simulink model "Mecanum_Mfunction_SM"  (R2022b)
settings: Solver=FixedStepAuto  StartTime=0.0  StopTime=20  FixedStep=0.001  RelTol=1e-3
values from neighbouring files (symbols this model uses):
  Cm = 0    [Mecanum_parameter_Mfunction_PI.m]    (also in Mecanum_parameter_Mfunction_PID.m; Mecanum_parameter_Mfunction_SM.m)
  Jm = 0    [Mecanum_parameter_Mfunction_PI.m]    (also in Mecanum_parameter_Mfunction_PID.m = 1.55e-06; Mecanum_parameter_Mfunction_SM.m)
  Kb = Kt    (= 230)    [Mecanum_parameter_Mfunction_PI.m]    (also in Mecanum_parameter_Mfunction_PID.m; Mecanum_parameter_Mfunction_SM.m)
  Kf = 0    [Mecanum_parameter_Mfunction_PI.m]    (also in Mecanum_parameter_Mfunction_PID.m; Mecanum_parameter_Mfunction_SM.m)
  Kt = 230    [Mecanum_parameter_Mfunction_PI.m]    (also in Mecanum_parameter_Mfunction_PID.m; Mecanum_parameter_Mfunction_SM.m)
  La = 0.39*10^-3    (= 0.00039)    [Mecanum_parameter_Mfunction_PI.m]    (also in Mecanum_parameter_Mfunction_PID.m; Mecanum_parameter_Mfunction_SM.m)
  N = N_motor * N_wheel    (= 10)    [Mecanum_parameter_Mfunction_PI.m]    (also in Mecanum_parameter_Mfunction_PID.m; Mecanum_parameter_Mfunction_SM.m)
  Ra = 0.38    [Mecanum_parameter_Mfunction_PI.m]    (also in Mecanum_parameter_Mfunction_PID.m; Mecanum_parameter_Mfunction_SM.m)
libraries: simulink x2
settings Model: Creator=HONG  LastModifiedBy=CSPLAB
settings SolverCC: AlgebraicLoopSolver=TrustRegion
settings DataIOCC: ReturnWorkspaceOutputs=off
settings DebuggingCC: UnconnectedInputMsg=warning  UnconnectedOutputMsg=warning  UnconnectedLineMsg=warning  SFMachineParentedDataDiag=warning  ArithmeticOperatorsInVariantConditions=warning
settings ModelReferenceCC: EnableRefExpFcnMdlSchedulingChecks=on
settings SFSimCC: CustomCodeUndefinedFunction=UseInterfaceOnly

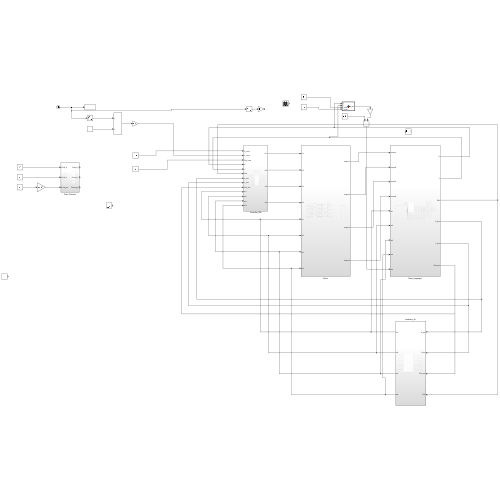
[thumbnail: Simulink's stored preview of the top-level diagram]
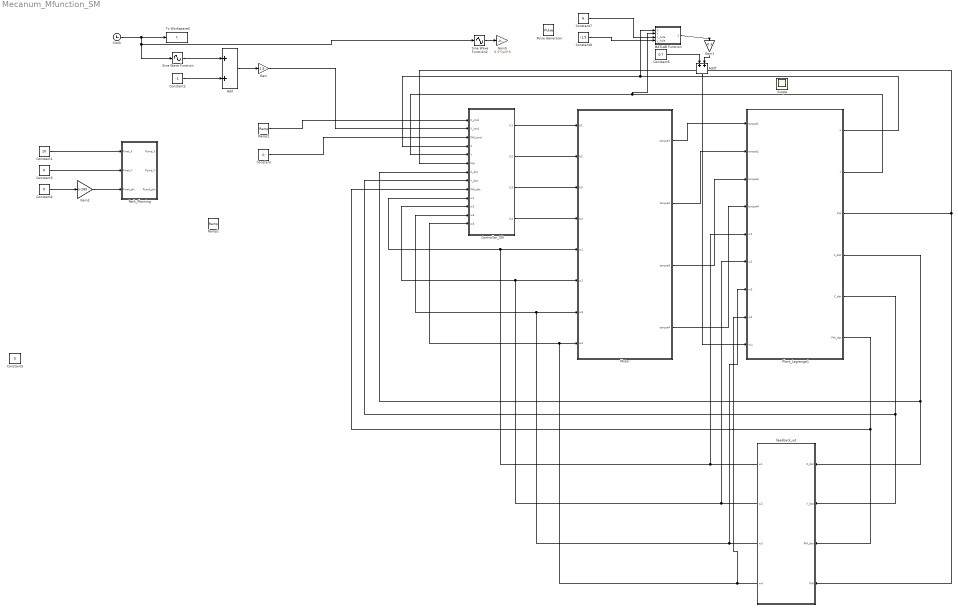
== system Mecanum_Mfunction_SM ==
  Add : Sum
  Add7 : Sum
  Clock : Clock
  Constant{,3..5} (4 alike) : Constant  Value=0
  Constant1 : Constant  Value=10
  Constant2 : Constant  Value=-1
  Constant6 : Constant  Value=0.7
  Constant7 : Constant  Value=6
  Constant8 : Constant  Value=-1.5
  Controller_SM : Subsystem
  Gain : Gain  Gain=1.5
  Gain1 : Gain  Gain=-0.3
  Gain2 : Gain  Gain=pi/180
  Gain5 : Gain  Gain=0.5*1e3*0
  MATLAB Function : MATLAB Function  TreatAsAtomicUnit=on
  Motor : Subsystem
  Path_Planning : Subsystem
  Plant_Lagrange1 : Subsystem
  Pulse Generator : DiscretePulseGenerator  PulseType=Time based  Period=10  PulseWidth=5
  Ramp1 : simulink/Sources/Ramp  slope=1.5  start=0  InitialOutput=0
  Ramp2 : simulink/Sources/Ramp  slope=0.5  start=0  InitialOutput=0
  Scope : Scope
  Sine Wave Function : Sin  TimeSource=Use external signal  Frequency=pi/8  Phase=pi/2  SampleTime=0
  Sine Wave Function2 : Sin  TimeSource=Use external signal  Frequency=pi/0.5  Phase=pi/2  SampleTime=0
  To Workspace5 : ToWorkspace  VariableName=t  SampleTime=-1
  feedback_w1 : Subsystem
  wires:
  Plant_Lagrange1/4(X_dot) -> Controller_SM/7(X_dot), feedback_w1/1(X_dot)
  Plant_Lagrange1/5(Y_dot) -> Controller_SM/8(Y_dot), feedback_w1/2(Y_dot)
  Plant_Lagrange1/6(PHI_dot) -> Controller_SM/9(PHI_dot), feedback_w1/3(PHI_dot)
  Plant_Lagrange1/3(PHI) -> feedback_w1/4(PHI), Controller_SM/6(PHI)
  feedback_w1/1(w1) -> Controller_SM/10(w1), Motor/5(w1), Plant_Lagrange1/5(w1)
  feedback_w1/2(w2) -> Plant_Lagrange1/6(w2), Controller_SM/11(w2), Motor/6(w2)
  feedback_w1/3(w3) -> Plant_Lagrange1/7(w3), Controller_SM/12(w3), Motor/7(w3)
  feedback_w1/4(w4) -> Plant_Lagrange1/8(w4), Controller_SM/13(w4), Motor/8(w4)
  Plant_Lagrange1/1(X) -> MATLAB Function/1(X), Controller_SM/4(X)
  Plant_Lagrange1/2(Y) -> MATLAB Function/2(Y), Controller_SM/5(Y)
  Clock/1 -> Sine Wave Function/1, Sine Wave Function2/1, To Workspace5/1
  Controller_SM/1(U1) -> Motor/1(U1)
  Controller_SM/2(U2) -> Motor/2(U2)
  Controller_SM/3(U3) -> Motor/3(U3)
  Controller_SM/4(U4) -> Motor/4(U4)
  Constant/1 -> Controller_SM/3(PHI_cmd)
  Constant2/1 -> Add/2
  Add/1 -> Gain/1
  Sine Wave Function/1 -> Add/1
  Constant1/1 -> Path_Planning/1(Final_X)
  Constant3/1 -> Path_Planning/2(Final_Y)
  Gain2/1 -> Path_Planning/3(Final_phi)
  Constant4/1 -> Gain2/1
  Gain/1 -> Controller_SM/2(Y_cmd)
  Ramp2/1 -> Controller_SM/1(X_cmd)
  Sine Wave Function2/1 -> Gain5/1
  Gain1/1 -> Add7/2
  Motor/2(torque2) -> Plant_Lagrange1/2(torque2)
  Motor/1(torque1) -> Plant_Lagrange1/1(torque1)
  Motor/3(torque3) -> Plant_Lagrange1/3(torque3)
  Motor/4(torque4) -> Plant_Lagrange1/4(torque4)
  Add7/1 -> Plant_Lagrange1/9(mu)
  Constant6/1 -> Add7/1
  MATLAB Function/1(Delta_mu) -> Gain1/1
  Constant7/1 -> MATLAB Function/3(x_hole)
  Constant8/1 -> MATLAB Function/4(y_hole)

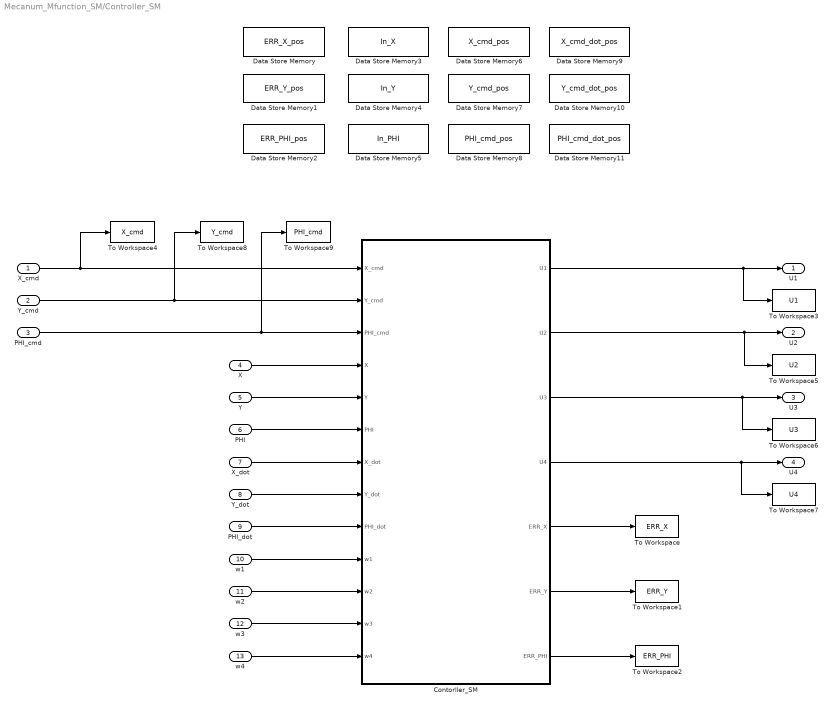
== system Mecanum_Mfunction_SM/Controller_SM ==
  X_cmd : Inport
  Y_cmd : Inport  Port=2
  PHI_cmd : Inport  Port=3
  X : Inport  Port=4
  Y : Inport  Port=5
  PHI : Inport  Port=6
  X_dot : Inport  Port=7
  Y_dot : Inport  Port=8
  PHI_dot : Inport  Port=9
  w1 : Inport  Port=10
  w2 : Inport  Port=11
  w3 : Inport  Port=12
  w4 : Inport  Port=13
  "Contorller_SM " : MATLAB Function  TreatAsAtomicUnit=on
  Data Store Memory : DataStoreMemory  DataStoreName=ERR_X_pos  ReadBeforeWriteMsg=warning  WriteAfterWriteMsg=warning  WriteAfterReadMsg=warning  ShowAdditionalParam=off  OutDataTypeStr=double
  Data Store Memory1 : DataStoreMemory  DataStoreName=ERR_Y_pos  ReadBeforeWriteMsg=warning  WriteAfterWriteMsg=warning  WriteAfterReadMsg=warning  ShowAdditionalParam=off  OutDataTypeStr=double
  Data Store Memory10 : DataStoreMemory  DataStoreName=Y_cmd_dot_pos  ReadBeforeWriteMsg=warning  WriteAfterWriteMsg=warning  WriteAfterReadMsg=warning  ShowAdditionalParam=off  OutDataTypeStr=double
  Data Store Memory11 : DataStoreMemory  DataStoreName=PHI_cmd_dot_pos  ReadBeforeWriteMsg=warning  WriteAfterWriteMsg=warning  WriteAfterReadMsg=warning  ShowAdditionalParam=off  OutDataTypeStr=double
  Data Store Memory2 : DataStoreMemory  DataStoreName=ERR_PHI_pos  ReadBeforeWriteMsg=warning  WriteAfterWriteMsg=warning  WriteAfterReadMsg=warning  ShowAdditionalParam=off  OutDataTypeStr=double
  Data Store Memory3 : DataStoreMemory  DataStoreName=In_X  ReadBeforeWriteMsg=warning  WriteAfterWriteMsg=warning  WriteAfterReadMsg=warning  ShowAdditionalParam=off  OutDataTypeStr=double
  Data Store Memory4 : DataStoreMemory  DataStoreName=In_Y  ReadBeforeWriteMsg=warning  WriteAfterWriteMsg=warning  WriteAfterReadMsg=warning  ShowAdditionalParam=off  OutDataTypeStr=double
  Data Store Memory5 : DataStoreMemory  DataStoreName=In_PHI  ReadBeforeWriteMsg=warning  WriteAfterWriteMsg=warning  WriteAfterReadMsg=warning  ShowAdditionalParam=off  OutDataTypeStr=double
  Data Store Memory6 : DataStoreMemory  DataStoreName=X_cmd_pos  ReadBeforeWriteMsg=warning  WriteAfterWriteMsg=warning  WriteAfterReadMsg=warning  ShowAdditionalParam=off  OutDataTypeStr=double
  Data Store Memory7 : DataStoreMemory  DataStoreName=Y_cmd_pos  ReadBeforeWriteMsg=warning  WriteAfterWriteMsg=warning  WriteAfterReadMsg=warning  ShowAdditionalParam=off  OutDataTypeStr=double
  Data Store Memory8 : DataStoreMemory  DataStoreName=PHI_cmd_pos  ReadBeforeWriteMsg=warning  WriteAfterWriteMsg=warning  WriteAfterReadMsg=warning  ShowAdditionalParam=off  OutDataTypeStr=double
  Data Store Memory9 : DataStoreMemory  DataStoreName=X_cmd_dot_pos  ReadBeforeWriteMsg=warning  WriteAfterWriteMsg=warning  WriteAfterReadMsg=warning  ShowAdditionalParam=off  OutDataTypeStr=double
  To Workspace : ToWorkspace  VariableName=ERR_X  SampleTime=-1
  To Workspace1 : ToWorkspace  VariableName=ERR_Y  SampleTime=-1
  To Workspace2 : ToWorkspace  VariableName=ERR_PHI  SampleTime=-1
  To Workspace3 : ToWorkspace  VariableName=U1  SampleTime=-1
  To Workspace4 : ToWorkspace  VariableName=X_cmd  SampleTime=-1
  To Workspace5 : ToWorkspace  VariableName=U2  SampleTime=-1
  To Workspace6 : ToWorkspace  VariableName=U3  SampleTime=-1
  To Workspace7 : ToWorkspace  VariableName=U4  SampleTime=-1
  To Workspace8 : ToWorkspace  VariableName=Y_cmd  SampleTime=-1
  To Workspace9 : ToWorkspace  VariableName=PHI_cmd  SampleTime=-1
  U1 : Outport  VectorParamsAs1DForOutWhenUnconnected=off
  U2 : Outport  Port=2  VectorParamsAs1DForOutWhenUnconnected=off
  U3 : Outport  Port=3  VectorParamsAs1DForOutWhenUnconnected=off
  U4 : Outport  Port=4  VectorParamsAs1DForOutWhenUnconnected=off
  wires:
  "Contorller_SM "/4(U4) -> To Workspace7/1, U4/1
  "Contorller_SM "/3(U3) -> To Workspace6/1, U3/1
  "Contorller_SM "/2(U2) -> To Workspace5/1, U2/1
  "Contorller_SM "/1(U1) -> U1/1, To Workspace3/1
  w4/1 -> "Contorller_SM "/13(w4)
  w3/1 -> "Contorller_SM "/12(w3)
  w2/1 -> "Contorller_SM "/11(w2)
  w1/1 -> "Contorller_SM "/10(w1)
  PHI_dot/1 -> "Contorller_SM "/9(PHI_dot)
  Y_dot/1 -> "Contorller_SM "/8(Y_dot)
  X_dot/1 -> "Contorller_SM "/7(X_dot)
  PHI/1 -> "Contorller_SM "/6(PHI)
  Y/1 -> "Contorller_SM "/5(Y)
  X/1 -> "Contorller_SM "/4(X)
  PHI_cmd/1 -> To Workspace9/1, "Contorller_SM "/3(PHI_cmd)
  Y_cmd/1 -> To Workspace8/1, "Contorller_SM "/2(Y_cmd)
  X_cmd/1 -> To Workspace4/1, "Contorller_SM "/1(X_cmd)
  "Contorller_SM "/5(ERR_X) -> To Workspace/1
  "Contorller_SM "/7(ERR_PHI) -> To Workspace2/1
  "Contorller_SM "/6(ERR_Y) -> To Workspace1/1

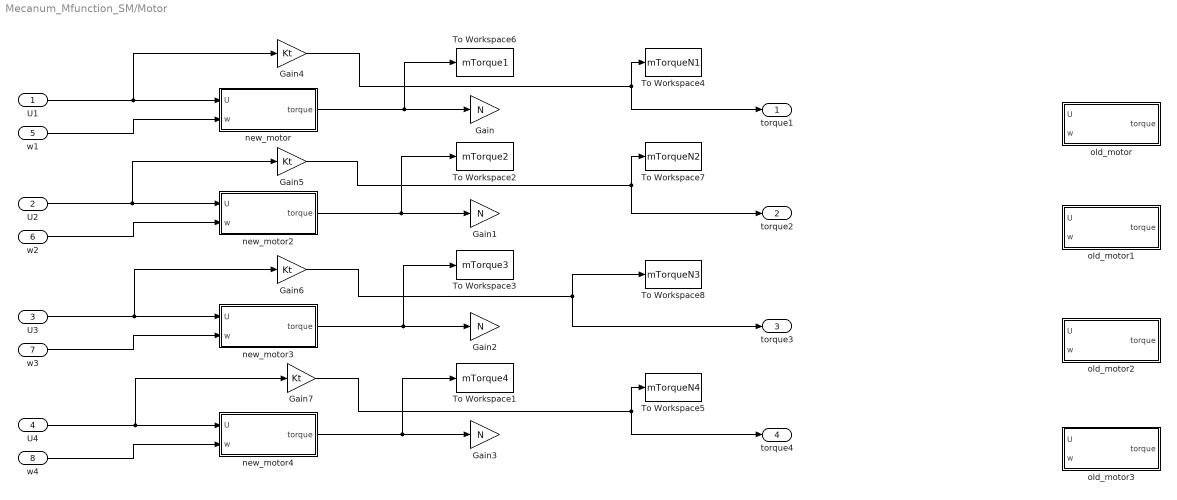
== system Mecanum_Mfunction_SM/Motor ==
  U1 : Inport
  U2 : Inport  Port=2
  U3 : Inport  Port=3
  U4 : Inport  Port=4
  w1 : Inport  Port=5
  w2 : Inport  Port=6
  w3 : Inport  Port=7
  w4 : Inport  Port=8
  Gain{,1..3} (4 alike) : Gain  Gain=N
  Gain{4..7} (4 alike) : Gain  Gain=Kt
  To Workspace1 : ToWorkspace  VariableName=mTorque4  SampleTime=-1
  To Workspace2 : ToWorkspace  VariableName=mTorque2  SampleTime=-1
  To Workspace3 : ToWorkspace  VariableName=mTorque3  SampleTime=-1
  To Workspace4 : ToWorkspace  VariableName=mTorqueN1  SampleTime=-1
  To Workspace5 : ToWorkspace  VariableName=mTorqueN4  SampleTime=-1
  To Workspace6 : ToWorkspace  VariableName=mTorque1  SampleTime=-1
  To Workspace7 : ToWorkspace  VariableName=mTorqueN2  SampleTime=-1
  To Workspace8 : ToWorkspace  VariableName=mTorqueN3  SampleTime=-1
  new_motor : Subsystem
  new_motor2 : Subsystem
  new_motor3 : Subsystem
  new_motor4 : Subsystem
  old_motor : Subsystem
  old_motor1 : Subsystem
  old_motor2 : Subsystem
  old_motor3 : Subsystem
  torque1 : Outport  VectorParamsAs1DForOutWhenUnconnected=off
  torque2 : Outport  Port=2  VectorParamsAs1DForOutWhenUnconnected=off
  torque3 : Outport  Port=3  VectorParamsAs1DForOutWhenUnconnected=off
  torque4 : Outport  Port=4  VectorParamsAs1DForOutWhenUnconnected=off
  wires:
  U1/1 -> Gain4/1, new_motor/1(U)
  w1/1 -> new_motor/2(w)
  w2/1 -> new_motor2/2(w)
  U2/1 -> Gain5/1, new_motor2/1(U)
  U3/1 -> Gain6/1, new_motor3/1(U)
  w3/1 -> new_motor3/2(w)
  U4/1 -> Gain7/1, new_motor4/1(U)
  w4/1 -> new_motor4/2(w)
  new_motor/1(torque) -> To Workspace6/1, Gain/1
  new_motor2/1(torque) -> To Workspace2/1, Gain1/1
  new_motor3/1(torque) -> To Workspace3/1, Gain2/1
  new_motor4/1(torque) -> Gain3/1, To Workspace1/1
  Gain4/1 -> To Workspace4/1, torque1/1
  Gain7/1 -> To Workspace5/1, torque4/1
  Gain6/1 -> To Workspace8/1, torque3/1
  Gain5/1 -> To Workspace7/1, torque2/1

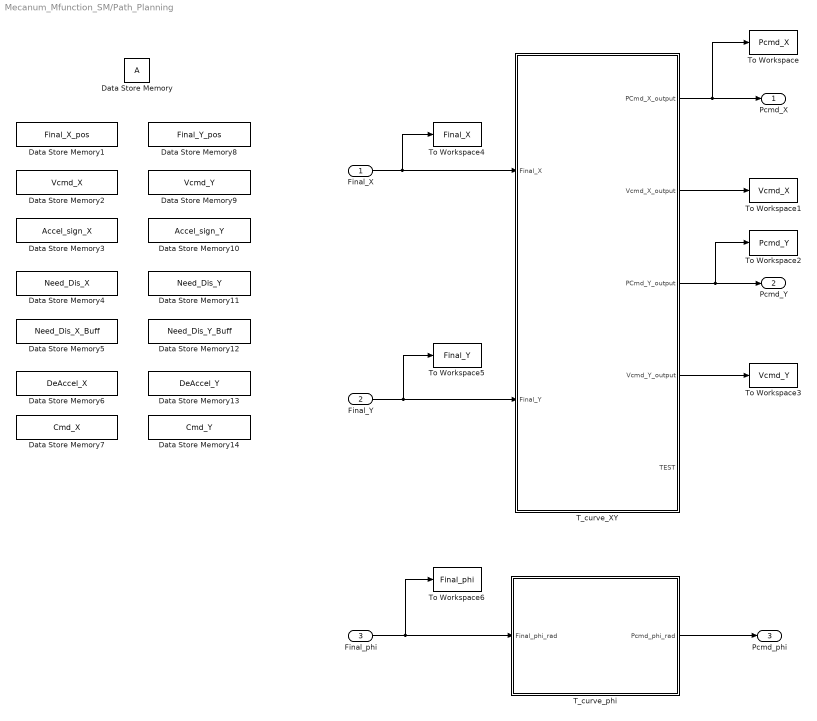
== system Mecanum_Mfunction_SM/Path_Planning ==
  Final_X : Inport
  Final_Y : Inport  Port=2
  Final_phi : Inport  Port=3
  Data Store Memory : DataStoreMemory  ReadBeforeWriteMsg=warning  WriteAfterWriteMsg=warning  WriteAfterReadMsg=warning  ShowAdditionalParam=off  OutDataTypeStr=double
  Data Store Memory1 : DataStoreMemory  DataStoreName=Final_X_pos  ReadBeforeWriteMsg=warning  WriteAfterWriteMsg=warning  WriteAfterReadMsg=warning  ShowAdditionalParam=off  OutDataTypeStr=double
  Data Store Memory10 : DataStoreMemory  DataStoreName=Accel_sign_Y  ReadBeforeWriteMsg=warning  WriteAfterWriteMsg=warning  WriteAfterReadMsg=warning  ShowAdditionalParam=off  OutDataTypeStr=double
  Data Store Memory11 : DataStoreMemory  DataStoreName=Need_Dis_Y  ReadBeforeWriteMsg=warning  WriteAfterWriteMsg=warning  WriteAfterReadMsg=warning  ShowAdditionalParam=off  OutDataTypeStr=double
  Data Store Memory12 : DataStoreMemory  DataStoreName=Need_Dis_Y_Buff  ReadBeforeWriteMsg=warning  WriteAfterWriteMsg=warning  WriteAfterReadMsg=warning  ShowAdditionalParam=off  OutDataTypeStr=double
  Data Store Memory13 : DataStoreMemory  DataStoreName=DeAccel_Y  ReadBeforeWriteMsg=warning  WriteAfterWriteMsg=warning  WriteAfterReadMsg=warning  ShowAdditionalParam=off  OutDataTypeStr=double
  Data Store Memory14 : DataStoreMemory  DataStoreName=Cmd_Y  ReadBeforeWriteMsg=warning  WriteAfterWriteMsg=warning  WriteAfterReadMsg=warning  ShowAdditionalParam=off  OutDataTypeStr=double
  Data Store Memory2 : DataStoreMemory  DataStoreName=Vcmd_X  ReadBeforeWriteMsg=warning  WriteAfterWriteMsg=warning  WriteAfterReadMsg=warning  ShowAdditionalParam=off  OutDataTypeStr=double
  Data Store Memory3 : DataStoreMemory  DataStoreName=Accel_sign_X  ReadBeforeWriteMsg=warning  WriteAfterWriteMsg=warning  WriteAfterReadMsg=warning  ShowAdditionalParam=off  OutDataTypeStr=double
  Data Store Memory4 : DataStoreMemory  DataStoreName=Need_Dis_X  ReadBeforeWriteMsg=warning  WriteAfterWriteMsg=warning  WriteAfterReadMsg=warning  ShowAdditionalParam=off  OutDataTypeStr=double
  Data Store Memory5 : DataStoreMemory  DataStoreName=Need_Dis_X_Buff  ReadBeforeWriteMsg=warning  WriteAfterWriteMsg=warning  WriteAfterReadMsg=warning  ShowAdditionalParam=off  OutDataTypeStr=double
  Data Store Memory6 : DataStoreMemory  DataStoreName=DeAccel_X  ReadBeforeWriteMsg=warning  WriteAfterWriteMsg=warning  WriteAfterReadMsg=warning  ShowAdditionalParam=off  OutDataTypeStr=double
  Data Store Memory7 : DataStoreMemory  DataStoreName=Cmd_X  ReadBeforeWriteMsg=warning  WriteAfterWriteMsg=warning  WriteAfterReadMsg=warning  ShowAdditionalParam=off  OutDataTypeStr=double
  Data Store Memory8 : DataStoreMemory  DataStoreName=Final_Y_pos  ReadBeforeWriteMsg=warning  WriteAfterWriteMsg=warning  WriteAfterReadMsg=warning  ShowAdditionalParam=off  OutDataTypeStr=double
  Data Store Memory9 : DataStoreMemory  DataStoreName=Vcmd_Y  ReadBeforeWriteMsg=warning  WriteAfterWriteMsg=warning  WriteAfterReadMsg=warning  ShowAdditionalParam=off  OutDataTypeStr=double
  "T_curve_XY " : MATLAB Function  TreatAsAtomicUnit=on
  T_curve_phi : Subsystem
  To Workspace : ToWorkspace  VariableName=Pcmd_X  SampleTime=-1
  To Workspace1 : ToWorkspace  VariableName=Vcmd_X  SampleTime=-1
  To Workspace2 : ToWorkspace  VariableName=Pcmd_Y  SampleTime=-1
  To Workspace3 : ToWorkspace  VariableName=Vcmd_Y  SampleTime=-1
  To Workspace4 : ToWorkspace  VariableName=Final_X  SampleTime=-1
  To Workspace5 : ToWorkspace  VariableName=Final_Y  SampleTime=-1
  To Workspace6 : ToWorkspace  VariableName=Final_phi  SampleTime=-1
  Pcmd_X : Outport  VectorParamsAs1DForOutWhenUnconnected=off
  Pcmd_Y : Outport  Port=2  VectorParamsAs1DForOutWhenUnconnected=off
  Pcmd_phi : Outport  Port=3  VectorParamsAs1DForOutWhenUnconnected=off
  wires:
  Final_X/1 -> To Workspace4/1, "T_curve_XY "/1(Final_X)
  Final_Y/1 -> To Workspace5/1, "T_curve_XY "/2(Final_Y)
  "T_curve_XY "/1(PCmd_X_output) -> To Workspace/1, Pcmd_X/1
  "T_curve_XY "/3(PCmd_Y_output) -> To Workspace2/1, Pcmd_Y/1
  "T_curve_XY "/2(Vcmd_X_output) -> To Workspace1/1
  "T_curve_XY "/4(Vcmd_Y_output) -> To Workspace3/1
  Final_phi/1 -> To Workspace6/1, T_curve_phi/1(Final_phi_rad)
  T_curve_phi/1(Pcmd_phi_rad) -> Pcmd_phi/1

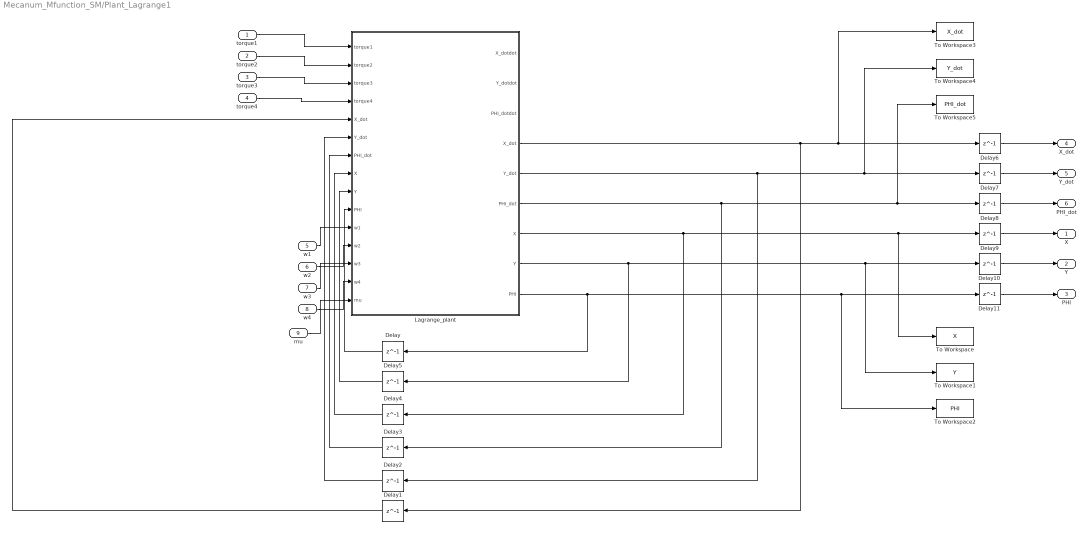
== system Mecanum_Mfunction_SM/Plant_Lagrange1 ==
  torque1 : Inport
  torque2 : Inport  Port=2
  torque3 : Inport  Port=3
  torque4 : Inport  Port=4
  w1 : Inport  Port=5
  w2 : Inport  Port=6
  w3 : Inport  Port=7
  w4 : Inport  Port=8
  mu : Inport  Port=9
  Delay{,1..11} (12 alike) : Delay  DelayLength=1  InitialCondition=0
  "Lagrange_plant " : MATLAB Function  TreatAsAtomicUnit=on
  To Workspace : ToWorkspace  VariableName=X  SampleTime=-1
  To Workspace1 : ToWorkspace  VariableName=Y  SampleTime=-1
  To Workspace2 : ToWorkspace  VariableName=PHI  SampleTime=-1
  To Workspace3 : ToWorkspace  VariableName=X_dot  SampleTime=-1
  To Workspace4 : ToWorkspace  VariableName=Y_dot  SampleTime=-1
  To Workspace5 : ToWorkspace  VariableName=PHI_dot  SampleTime=-1
  X : Outport  VectorParamsAs1DForOutWhenUnconnected=off
  Y : Outport  Port=2  VectorParamsAs1DForOutWhenUnconnected=off
  PHI : Outport  Port=3  VectorParamsAs1DForOutWhenUnconnected=off
  X_dot : Outport  Port=4  VectorParamsAs1DForOutWhenUnconnected=off
  Y_dot : Outport  Port=5  VectorParamsAs1DForOutWhenUnconnected=off
  PHI_dot : Outport  Port=6  VectorParamsAs1DForOutWhenUnconnected=off
  wires:
  "Lagrange_plant "/9(PHI) -> Delay/1, To Workspace2/1, Delay11/1
  "Lagrange_plant "/8(Y) -> Delay5/1, To Workspace1/1, Delay10/1
  "Lagrange_plant "/7(X) -> Delay4/1, To Workspace/1, Delay9/1
  "Lagrange_plant "/6(PHI_dot) -> Delay3/1, To Workspace5/1, Delay8/1
  "Lagrange_plant "/5(Y_dot) -> Delay2/1, To Workspace4/1, Delay7/1
  "Lagrange_plant "/4(X_dot) -> Delay1/1, To Workspace3/1, Delay6/1
  Delay2/1 -> "Lagrange_plant "/6("Y_dot ")
  Delay1/1 -> "Lagrange_plant "/5("X_dot ")
  torque1/1 -> "Lagrange_plant "/1(torque1)
  torque2/1 -> "Lagrange_plant "/2(torque2)
  torque3/1 -> "Lagrange_plant "/3(torque3)
  torque4/1 -> "Lagrange_plant "/4(torque4)
  Delay/1 -> "Lagrange_plant "/10("PHI ")
  Delay5/1 -> "Lagrange_plant "/9("Y ")
  Delay4/1 -> "Lagrange_plant "/8("X ")
  Delay3/1 -> "Lagrange_plant "/7("PHI_dot ")
  Delay6/1 -> X_dot/1
  Delay7/1 -> Y_dot/1
  Delay8/1 -> PHI_dot/1
  Delay9/1 -> X/1
  Delay10/1 -> Y/1
  Delay11/1 -> PHI/1
  w4/1 -> "Lagrange_plant "/14(w4)
  w3/1 -> "Lagrange_plant "/13(w3)
  w2/1 -> "Lagrange_plant "/12(w2)
  w1/1 -> "Lagrange_plant "/11(w1)
  mu/1 -> "Lagrange_plant "/15(mu)

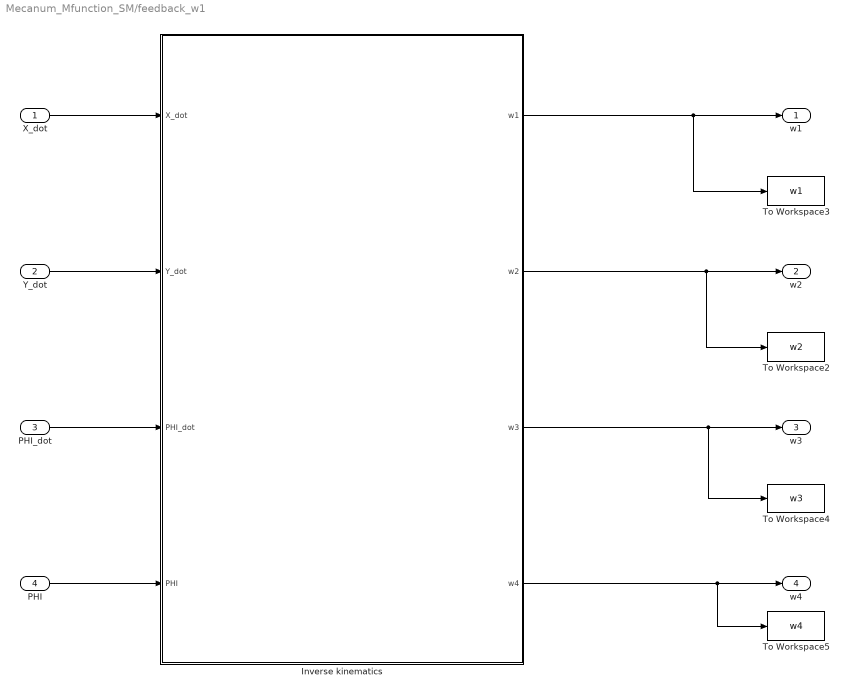
== system Mecanum_Mfunction_SM/feedback_w1 ==
  X_dot : Inport
  Y_dot : Inport  Port=2
  PHI_dot : Inport  Port=3
  PHI : Inport  Port=4
  "Inverse kinematics " : MATLAB Function  TreatAsAtomicUnit=on
  To Workspace2 : ToWorkspace  VariableName=w2  SampleTime=-1
  To Workspace3 : ToWorkspace  VariableName=w1  SampleTime=-1
  To Workspace4 : ToWorkspace  VariableName=w3  SampleTime=-1
  To Workspace5 : ToWorkspace  VariableName=w4  SampleTime=-1
  w1 : Outport  VectorParamsAs1DForOutWhenUnconnected=off
  w2 : Outport  Port=2  VectorParamsAs1DForOutWhenUnconnected=off
  w3 : Outport  Port=3  VectorParamsAs1DForOutWhenUnconnected=off
  w4 : Outport  Port=4  VectorParamsAs1DForOutWhenUnconnected=off
  wires:
  PHI_dot/1 -> "Inverse kinematics "/3(PHI_dot)
  PHI/1 -> "Inverse kinematics "/4(PHI)
  Y_dot/1 -> "Inverse kinematics "/2(Y_dot)
  X_dot/1 -> "Inverse kinematics "/1(X_dot)
  "Inverse kinematics "/1(w1) -> To Workspace3/1, w1/1
  "Inverse kinematics "/2(w2) -> To Workspace2/1, w2/1
  "Inverse kinematics "/3(w3) -> To Workspace4/1, w3/1
  "Inverse kinematics "/4(w4) -> To Workspace5/1, w4/1

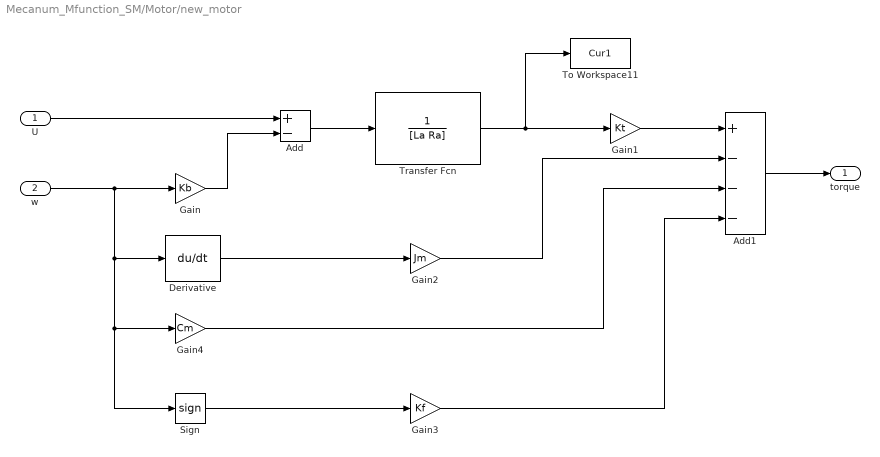
== system Mecanum_Mfunction_SM/Motor/new_motor ==
  U : Inport
  w : Inport  Port=2
  Add : Sum  Inputs=+-
  Add1 : Sum  Inputs=+---
  Derivative : Derivative
  Gain : Gain  Gain=Kb
  Gain1 : Gain  Gain=Kt
  Gain2 : Gain  Gain=Jm
  Gain3 : Gain  Gain=Kf
  Gain4 : Gain  Gain=Cm
  Sign : Signum  ZeroCross=off
  To Workspace11 : ToWorkspace  VariableName=Cur1  SampleTime=-1
  Transfer Fcn : TransferFcn  Denominator=[La Ra]
  torque : Outport  VectorParamsAs1DForOutWhenUnconnected=off
  wires:
  Add1/1 -> torque/1
  Gain2/1 -> Add1/2
  Derivative/1 -> Gain2/1
  Gain1/1 -> Add1/1
  Gain4/1 -> Add1/3
  Gain/1 -> Add/2
  Transfer Fcn/1 -> To Workspace11/1, Gain1/1
  Sign/1 -> Gain3/1
  w/1 -> Sign/1, Gain4/1, Derivative/1, Gain/1
  U/1 -> Add/1
  Gain3/1 -> Add1/4
  Add/1 -> Transfer Fcn/1

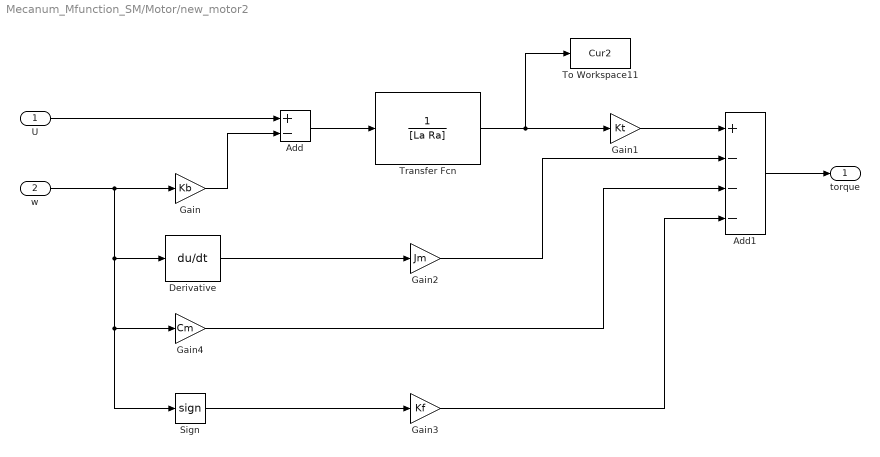
== system Mecanum_Mfunction_SM/Motor/new_motor2 ==
  U : Inport
  w : Inport  Port=2
  Add : Sum  Inputs=+-
  Add1 : Sum  Inputs=+---
  Derivative : Derivative
  Gain : Gain  Gain=Kb
  Gain1 : Gain  Gain=Kt
  Gain2 : Gain  Gain=Jm
  Gain3 : Gain  Gain=Kf
  Gain4 : Gain  Gain=Cm
  Sign : Signum  ZeroCross=off
  To Workspace11 : ToWorkspace  VariableName=Cur2  SampleTime=-1
  Transfer Fcn : TransferFcn  Denominator=[La Ra]
  torque : Outport  VectorParamsAs1DForOutWhenUnconnected=off
  wires:
  Add1/1 -> torque/1
  Gain2/1 -> Add1/2
  Derivative/1 -> Gain2/1
  Gain1/1 -> Add1/1
  Gain4/1 -> Add1/3
  Add/1 -> Transfer Fcn/1
  Gain/1 -> Add/2
  Transfer Fcn/1 -> To Workspace11/1, Gain1/1
  Sign/1 -> Gain3/1
  w/1 -> Sign/1, Gain4/1, Derivative/1, Gain/1
  U/1 -> Add/1
  Gain3/1 -> Add1/4

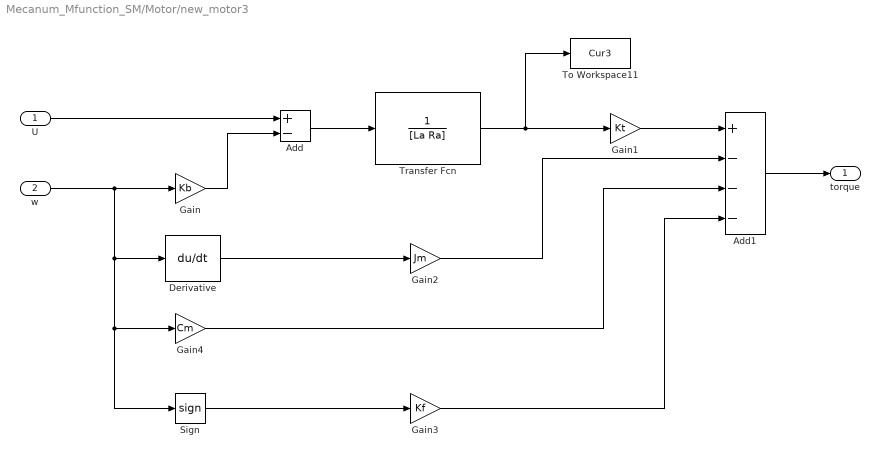
== system Mecanum_Mfunction_SM/Motor/new_motor3 ==
  U : Inport
  w : Inport  Port=2
  Add : Sum  Inputs=+-
  Add1 : Sum  Inputs=+---
  Derivative : Derivative
  Gain : Gain  Gain=Kb
  Gain1 : Gain  Gain=Kt
  Gain2 : Gain  Gain=Jm
  Gain3 : Gain  Gain=Kf
  Gain4 : Gain  Gain=Cm
  Sign : Signum  ZeroCross=off
  To Workspace11 : ToWorkspace  VariableName=Cur3  SampleTime=-1
  Transfer Fcn : TransferFcn  Denominator=[La Ra]
  torque : Outport  VectorParamsAs1DForOutWhenUnconnected=off
  wires:
  Add1/1 -> torque/1
  Gain2/1 -> Add1/2
  Derivative/1 -> Gain2/1
  Gain1/1 -> Add1/1
  Gain4/1 -> Add1/3
  Add/1 -> Transfer Fcn/1
  Gain/1 -> Add/2
  Transfer Fcn/1 -> To Workspace11/1, Gain1/1
  Sign/1 -> Gain3/1
  w/1 -> Sign/1, Gain4/1, Derivative/1, Gain/1
  U/1 -> Add/1
  Gain3/1 -> Add1/4

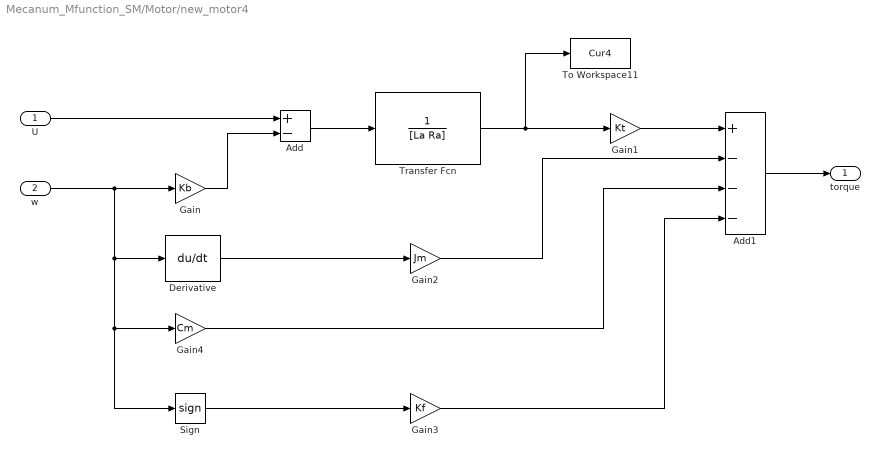
== system Mecanum_Mfunction_SM/Motor/new_motor4 ==
  U : Inport
  w : Inport  Port=2
  Add : Sum  Inputs=+-
  Add1 : Sum  Inputs=+---
  Derivative : Derivative
  Gain : Gain  Gain=Kb
  Gain1 : Gain  Gain=Kt
  Gain2 : Gain  Gain=Jm
  Gain3 : Gain  Gain=Kf
  Gain4 : Gain  Gain=Cm
  Sign : Signum  ZeroCross=off
  To Workspace11 : ToWorkspace  VariableName=Cur4  SampleTime=-1
  Transfer Fcn : TransferFcn  Denominator=[La Ra]
  torque : Outport  VectorParamsAs1DForOutWhenUnconnected=off
  wires:
  Add1/1 -> torque/1
  Gain2/1 -> Add1/2
  Derivative/1 -> Gain2/1
  Gain1/1 -> Add1/1
  Gain4/1 -> Add1/3
  Add/1 -> Transfer Fcn/1
  Gain/1 -> Add/2
  Transfer Fcn/1 -> To Workspace11/1, Gain1/1
  Sign/1 -> Gain3/1
  w/1 -> Sign/1, Gain4/1, Derivative/1, Gain/1
  U/1 -> Add/1
  Gain3/1 -> Add1/4

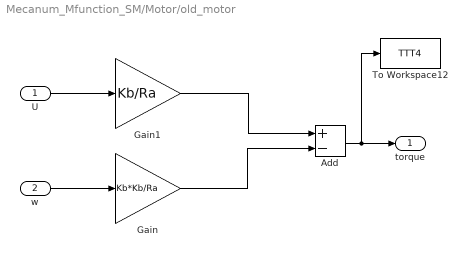
== system Mecanum_Mfunction_SM/Motor/old_motor ==
  U : Inport
  w : Inport  Port=2
  Add : Sum  Inputs=+-
  Gain : Gain  Gain=Kb*Kb/Ra
  Gain1 : Gain  Gain=Kb/Ra
  To Workspace12 : ToWorkspace  VariableName=TTT4  SampleTime=-1
  torque : Outport  VectorParamsAs1DForOutWhenUnconnected=off
  wires:
  U/1 -> Gain1/1
  w/1 -> Gain/1
  Gain1/1 -> Add/1
  Gain/1 -> Add/2
  Add/1 -> To Workspace12/1, torque/1

== system Mecanum_Mfunction_SM/Motor/old_motor1 ==
  U : Inport
  w : Inport  Port=2
  Add : Sum  Inputs=+-
  Gain : Gain  Gain=Kb*Kb/Ra
  Gain1 : Gain  Gain=Kb/Ra
  torque : Outport  VectorParamsAs1DForOutWhenUnconnected=off
  wires:
  U/1 -> Gain1/1
  w/1 -> Gain/1
  Gain1/1 -> Add/1
  Gain/1 -> Add/2
  Add/1 -> torque/1

== system Mecanum_Mfunction_SM/Motor/old_motor2 ==
  U : Inport
  w : Inport  Port=2
  Add : Sum  Inputs=+-
  Gain : Gain  Gain=Kb*Kb/Ra
  Gain1 : Gain  Gain=Kb/Ra
  torque : Outport  VectorParamsAs1DForOutWhenUnconnected=off
  wires:
  U/1 -> Gain1/1
  w/1 -> Gain/1
  Gain1/1 -> Add/1
  Gain/1 -> Add/2
  Add/1 -> torque/1

== system Mecanum_Mfunction_SM/Motor/old_motor3 ==
  U : Inport
  w : Inport  Port=2
  Add : Sum  Inputs=+-
  Gain : Gain  Gain=Kb*Kb/Ra
  Gain1 : Gain  Gain=Kb/Ra
  torque : Outport  VectorParamsAs1DForOutWhenUnconnected=off
  wires:
  U/1 -> Gain1/1
  w/1 -> Gain/1
  Gain1/1 -> Add/1
  Gain/1 -> Add/2
  Add/1 -> torque/1

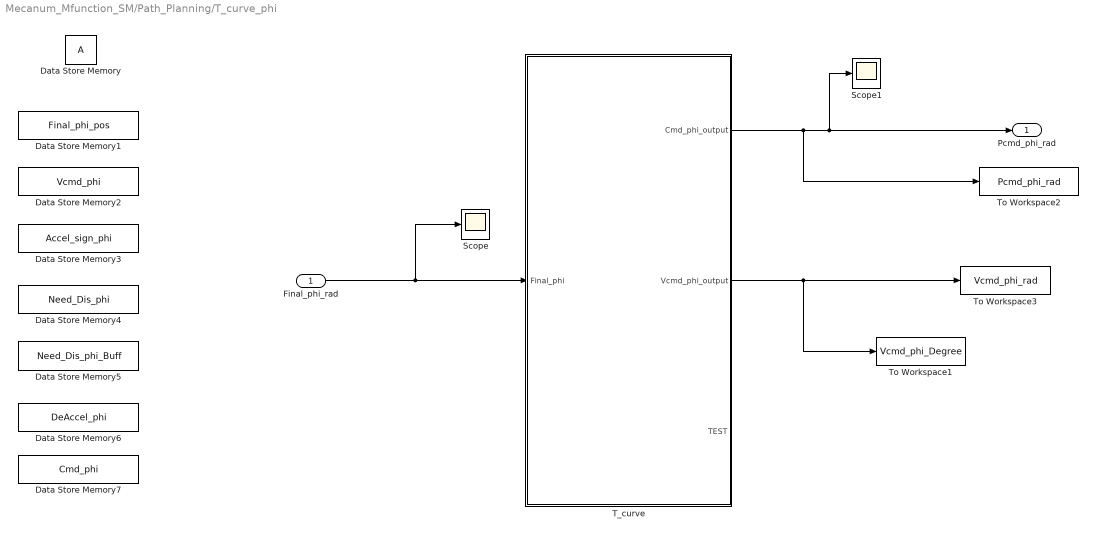
== system Mecanum_Mfunction_SM/Path_Planning/T_curve_phi ==
  Final_phi_rad : Inport
  Data Store Memory : DataStoreMemory  ReadBeforeWriteMsg=warning  WriteAfterWriteMsg=warning  WriteAfterReadMsg=warning  ShowAdditionalParam=off  OutDataTypeStr=double
  Data Store Memory1 : DataStoreMemory  DataStoreName=Final_phi_pos  ReadBeforeWriteMsg=warning  WriteAfterWriteMsg=warning  WriteAfterReadMsg=warning  ShowAdditionalParam=off  OutDataTypeStr=double
  Data Store Memory2 : DataStoreMemory  DataStoreName=Vcmd_phi  ReadBeforeWriteMsg=warning  WriteAfterWriteMsg=warning  WriteAfterReadMsg=warning  ShowAdditionalParam=off  OutDataTypeStr=double
  Data Store Memory3 : DataStoreMemory  DataStoreName=Accel_sign_phi  ReadBeforeWriteMsg=warning  WriteAfterWriteMsg=warning  WriteAfterReadMsg=warning  ShowAdditionalParam=off  OutDataTypeStr=double
  Data Store Memory4 : DataStoreMemory  DataStoreName=Need_Dis_phi  ReadBeforeWriteMsg=warning  WriteAfterWriteMsg=warning  WriteAfterReadMsg=warning  ShowAdditionalParam=off  OutDataTypeStr=double
  Data Store Memory5 : DataStoreMemory  DataStoreName=Need_Dis_phi_Buff  ReadBeforeWriteMsg=warning  WriteAfterWriteMsg=warning  WriteAfterReadMsg=warning  ShowAdditionalParam=off  OutDataTypeStr=double
  Data Store Memory6 : DataStoreMemory  DataStoreName=DeAccel_phi  ReadBeforeWriteMsg=warning  WriteAfterWriteMsg=warning  WriteAfterReadMsg=warning  ShowAdditionalParam=off  OutDataTypeStr=double
  Data Store Memory7 : DataStoreMemory  DataStoreName=Cmd_phi  ReadBeforeWriteMsg=warning  WriteAfterWriteMsg=warning  WriteAfterReadMsg=warning  ShowAdditionalParam=off  OutDataTypeStr=double
  Scope : Scope
  Scope1 : Scope
  T_curve : MATLAB Function  TreatAsAtomicUnit=on
  To Workspace1 : ToWorkspace  VariableName=Vcmd_phi_Degree  SampleTime=-1
  To Workspace2 : ToWorkspace  VariableName=Pcmd_phi_rad  SampleTime=-1
  To Workspace3 : ToWorkspace  VariableName=Vcmd_phi_rad  SampleTime=-1
  Pcmd_phi_rad : Outport  VectorParamsAs1DForOutWhenUnconnected=off
  wires:
  Final_phi_rad/1 -> T_curve/1(Final_phi), Scope/1
  T_curve/2(Vcmd_phi_output) -> To Workspace3/1, To Workspace1/1
  T_curve/1(Cmd_phi_output) -> Scope1/1, Pcmd_phi_rad/1, To Workspace2/1

== matlab function Mecanum_Mfunction_SM/Plant_Lagrange1/Lagrange_plant  ==
  settings: updateMethod=DISCRETE  sampleTime=0.001
  data: torque1 input; torque2 input; X_dotdot output; Y_dotdot output; PHI_dotdot output; torque3 input; torque4 input; X_dot input; Y_dot input; PHI_dot input; X input; Y input; PHI input; X_dot output; Y_dot output; PHI_dot output; X output; Y output; PHI output; w1 input; w2 input; w3 input; w4 input; mu input
function [X_dotdot,Y_dotdot,PHI_dotdot,X_dot,Y_dot,PHI_dot,X,Y,PHI]  = fcn(torque1,torque2,torque3,torque4,X_dot,Y_dot,PHI_dot,X,Y,PHI,w1,w2,w3,w4,mu)
%#codegen


%===== Parameter =====
%=== Body ===
mb = 480;   %Origin 10; Empty 320; Full 480; 
d = 1.18;   %0.6;
w = 0.85;  %0.4;
Izb = 1/12*mb*(d^2+w^2);

%=== Wheel ===
mw = 5.692; %0.4;
R = 0.127;  %0.05;
Iyw = mw*R^2/2;
Lx = 0.425; %0.2375;
Ly = 0.266; %0.2394;
Izw = mw*(Lx^2+Ly^2);

%=== Friction ====
Friction = (mb+4*mw)/4*9.8*mu;   % 0.4環氧樹脂 0.7磨石子地板

if(w1>1)
    torque1 = torque1 - Friction;
elseif(w1<-1)
    torque1 = torque1 + Friction;
end

if(w2>1)
    torque2 = torque2 - Friction;
elseif(w2<-1)
    torque2 = torque2 + Friction;
end

if(w3>1)
    torque3 = torque3 - Friction;
elseif(w3<-1)
    torque3 = torque3 + Friction;
end

if(w4>1)
    torque4 = torque4 - Friction;
elseif(w4<-1)
    torque4 = torque4 + Friction;
end

%% 懸空
% 馬達位置
Pos1 = [(X + Lx), (Y + Ly)];
Pos2 = [(X + Lx), (Y - Ly)];
Pos3 = [(X - Lx), (Y + Ly)];
Pos4 = [(X - Lx), (Y - Ly)];
Dist1 = ((Pos1(1) - 2)^2 + (Pos1(2) + 1.5)^2)^0.5;
Dist2 = ((Pos2(1) - 2)^2 + (Pos2(2) + 1.5)^2)^0.5;
Dist3 = ((Pos3(1) - 2)^2 + (Pos3(2) + 1.5)^2)^0.5;
Dist4 = ((Pos4(1) - 2)^2 + (Pos4(2) + 1.5)^2)^0.5;
if(Dist1 < 1)
    torque1 = 0;
end
% if(Dist2 < 0.5)
%     torque2 = 0;
% end
% if(Dist3 < 0.5)
%     torque3 = 0;
% end
% if(Dist4 < 0.5)
%     torque4 = 0;
% end

%%

dt = 0.001;

Den_XY  = mb + 4*mw + 4*(Iyw/(R^2));
Den_PHI = Izb + 4*Izw + 4*mw*(Lx^2+Ly^2) + 4*Iyw/(R^2)*(Lx+Ly)^2 ;

Buff_X   = (cos(PHI)+sin(PHI))/R*(torque1+torque4) + (cos(PHI)-sin(PHI))/R*(torque2+torque3) - 4*Iyw/(R^2)*Y_dot*PHI_dot;
Buff_Y   = (sin(PHI)-cos(PHI))/R*(torque1+torque4) + (sin(PHI)+cos(PHI))/R*(torque2+torque3) + 4*Iyw/(R^2)*X_dot*PHI_dot;
Buff_PHI = (Lx+Ly)/R*(-torque1+torque2-torque3+torque4);

X_dotdot   = Buff_X/Den_XY;
Y_dotdot   = Buff_Y/Den_XY;
PHI_dotdot = Buff_PHI/Den_PHI;


X_dot   = X_dot   + X_dotdot   *dt;
Y_dot   = Y_dot   + Y_dotdot   *dt;
PHI_dot = PHI_dot + PHI_dotdot *dt;

X   = X   + X_dot   *dt;
Y   = Y   + Y_dot   *dt;
PHI = PHI + PHI_dot *dt;

== matlab function Mecanum_Mfunction_SM/Path_Planning/T_curve_XY  ==
  settings: updateMethod=DISCRETE  sampleTime=0.001
  data: A data_store_memory; PCmd_X_output output; Vcmd_X_output output; PCmd_Y_output output; Vcmd_Y_output output; Final_X input; TEST output; Final_X_pos data_store_memory; Vcmd_X data_store_memory; Accel_sign_X data_store_memory; Need_Dis_X data_store_memory; Need_Dis_X_Buff data_store_memory; DeAccel_X data_store_memory; Cmd_X data_store_memory; Final_Y input; Vcmd_Y data_store_memory; Final_Y_pos data_store_memory; Accel_sign_Y data_store_memory; Need_Dis_Y data_store_memory; Need_Dis_Y_Buff data_store_memory; DeAccel_Y data_store_memory; Cmd_Y data_store_memory
function [PCmd_X_output,Vcmd_X_output,PCmd_Y_output,Vcmd_Y_output,TEST]    = fcn(Final_X,Final_Y)

%==== Ver 2 =====
global A;
global Final_X_pos;
global Final_Y_pos;
global Vcmd_X;
global Vcmd_Y;
global Accel_sign_X;
global Accel_sign_Y;
global Need_Dis_X;
global Need_Dis_Y;
global Need_Dis_X_Buff;
global Need_Dis_Y_Buff;
global DeAccel_X;
global DeAccel_Y;
global Cmd_X;
global Cmd_Y;

%===== Parameter=====
Max_Accel = 1;
Max_Velocity = 2;
Pos_Standard = 0.1;
dt = 0.001;

%=== CHECK Final Change? ===
if(Final_X ~= Final_X_pos)
    Need_Dis_X = Final_X - Cmd_X;
    Need_Dis_X_Buff =0;
    DeAccel_X =0;
    
    %=== Direction Check ===
	if (Need_Dis_X >0)
        Accel_sign_X =  1;
	elseif (Need_Dis_X <0)
		Accel_sign_X = -1;
	else
		Accel_sign_X =  0;
	end
end

if(Final_Y ~= Final_Y_pos)
    Need_Dis_Y = Final_Y - Cmd_Y;
    Need_Dis_Y_Buff =0;
    DeAccel_Y =0;
    
    %=== Direction Check ===
	if (Need_Dis_Y >0)
        Accel_sign_Y =  1;
	elseif (Need_Dis_Y <0)
		Accel_sign_Y = -1;
	else
		Accel_sign_Y =  0;
	end
end

%===== Max Velocity Check =====
if( (abs(Need_Dis_X_Buff - Need_Dis_X ) > Pos_Standard) && (abs(Need_Dis_Y_Buff - Need_Dis_Y ) > Pos_Standard))
    Max_Velocity = 1.3;
else
    Max_Velocity = 2;
end



Detime_Y = abs(Vcmd_Y/Max_Accel);     
Detime_X = abs(Vcmd_X/Max_Accel);

%===== DeAccel Cehck =====
%===== X =====
     Buff = Need_Dis_X_Buff + Vcmd_X*Detime_X + 1/2*(-1*Accel_sign_X*Max_Accel)*Detime_X*Detime_X;
    
    if((Buff>Need_Dis_X) && (Accel_sign_X==1))
        DeAccel_X = 1;
    elseif ((Buff<Need_Dis_X) && (Accel_sign_X==-1))
        DeAccel_X = 1;
    else
        DeAccel_X = 0;
    end
%===== Y =====    
         Buff = Need_Dis_Y_Buff + Vcmd_Y*Detime_Y + 1/2*(-1*Accel_sign_Y*Max_Accel)*Detime_Y*Detime_Y;
    
    if((Buff>Need_Dis_Y) && (Accel_sign_Y==1))
        DeAccel_Y = 1;
    elseif ((Buff<Need_Dis_Y) && (Accel_sign_Y==-1))
        DeAccel_Y = 1;
    else
        DeAccel_Y = 0;
    end
    
%===== Vel Cal =====
%===== X =====
if(DeAccel_X ==0)
    Vcmd_X = Vcmd_X + Accel_sign_X * Max_Accel*dt;
elseif(DeAccel_X ==1) 
    Vcmd_X = Vcmd_X - Accel_sign_X * Max_Accel*dt;
    Buff = Vcmd_X *Accel_sign_X;
    if(Buff<0)
    Vcmd_X = 0;
    end
end
%===== Y =====
if(DeAccel_Y ==0)
    Vcmd_Y = Vcmd_Y + Accel_sign_Y * Max_Accel*dt;
elseif(DeAccel_Y ==1) 
    Vcmd_Y = Vcmd_Y - Accel_sign_Y * Max_Accel*dt;
    Buff = Vcmd_Y *Accel_sign_Y;
    if(Buff<0)
    Vcmd_Y = 0;
    end
end

%===== Max Vel Check =====
%=== X ===
if(Vcmd_X > Max_Velocity)
    Vcmd_X = Max_Velocity;
elseif (Vcmd_X < -Max_Velocity)
    Vcmd_X = -Max_Velocity;
end
%=== Y ===
if(Vcmd_Y > Max_Velocity)
    Vcmd_Y = Max_Velocity;
elseif (Vcmd_Y < -Max_Velocity)
    Vcmd_Y = -Max_Velocity;
end


Cmd_X = Cmd_X + Vcmd_X * dt;
Cmd_Y = Cmd_Y + Vcmd_Y * dt;

Need_Dis_X_Buff = Need_Dis_X_Buff + Vcmd_X*dt;
Need_Dis_Y_Buff = Need_Dis_Y_Buff + Vcmd_Y*dt;

Final_X_pos = Final_X;
Final_Y_pos = Final_Y;

%===== Output =====
PCmd_X_output  = Cmd_X;
PCmd_Y_output  = Cmd_Y;

Vcmd_X_output = Vcmd_X;
Vcmd_Y_output = Vcmd_Y;

A = A+1;
TEST =A;

== matlab function Mecanum_Mfunction_SM/feedback_w1/Inverse kinematics  ==
  settings: updateMethod=DISCRETE  sampleTime=0.001
  data: X_dot input; Y_dot input; PHI_dot input; w1 output; w2 output; w3 output; w4 output; PHI input
function [w1,w2,w3,w4]  = fcn(X_dot,Y_dot,PHI_dot,PHI)
%#codegen




% ===== Parameter =====

Lx = 0.425; %0.2375;
Ly = 0.266; %0.2394;
R  = 0.127; %0.05;
N  = 10;    %14;


Xm_dot =  cos(PHI)*X_dot + sin(PHI)*Y_dot;  
Ym_dot = -sin(PHI)*X_dot + cos(PHI)*Y_dot;


Buff_w1 = Xm_dot - Ym_dot - (Lx+Ly)*PHI_dot;
Buff_w2 = Xm_dot + Ym_dot + (Lx+Ly)*PHI_dot;
Buff_w3 = Xm_dot + Ym_dot - (Lx+Ly)*PHI_dot;
Buff_w4 = Xm_dot - Ym_dot + (Lx+Ly)*PHI_dot;





w1 =Buff_w1/R*N;
w2 =Buff_w2/R*N;
w3 =Buff_w3/R*N;
w4 =Buff_w4/R*N;

== matlab function Mecanum_Mfunction_SM/Controller_SM/Contorller_SM  ==
  settings: updateMethod=DISCRETE  sampleTime=0.001
  data: X_cmd input; U1 output; U2 output; U3 output; U4 output; Y_cmd input; PHI_cmd input; X input; Y input; PHI input; X_dot input; Y_dot input; PHI_dot input; w1 input; w2 input; w3 input; w4 input; ERR_X_pos data_store_memory; ERR_Y_pos data_store_memory; ERR_PHI_pos data_store_memory; In_X data_store_memory; In_Y data_store_memory; In_PHI data_store_memory; X_cmd_pos data_store_memory; Y_cmd_pos data_store_memory; PHI_cmd_pos data_store_memory; X_cmd_dot_pos data_store_memory; Y_cmd_dot_pos data_store_memory; PHI_cmd_dot_pos data_store_memory; ERR_X output; ERR_Y output; ERR_PHI output
function [U1,U2,U3,U4,ERR_X,ERR_Y,ERR_PHI]  = fcn(X_cmd,Y_cmd,PHI_cmd,X,Y,PHI,X_dot,Y_dot,PHI_dot,w1,w2,w3,w4)
%#codegen

global In_X
global In_Y
global In_PHI
global ERR_X_pos
global ERR_Y_pos
global ERR_PHI_pos
global X_cmd_pos
global Y_cmd_pos
global PHI_cmd_pos
global X_cmd_dot_pos
global Y_cmd_dot_pos
global PHI_cmd_dot_pos


%===== Parameter =====
%=== Body ===
mb = 400;   %30; 
d = 0.44;   %0.6;
w = 0.347;  %0.4;
Izb = 1/12*mb*(d^2+w^2);

%=== Wheel ===
mw = 5.692; %0.4;
R = 0.127;  %0.05;
Iyw = mw*R^2/2;
Lx = 0.85;  %0.2375;
Ly = 0.266; %0.2394;
Izw = mw*(Lx^2+Ly^2);
%=== Motor ===
Ra = 0.38;
Kt = 230;   %28.6*10^-3;
Kb = Kt;

%=== Gear ===
N = 10; %14;

%=== Sat ===
MaxU = 13.7*3;  %24;

dt = 0.001;


%===== Controller =====
K = 6000;
Sigma = -3000;

Slide_sat = 2.5; %50

ERR_X   = X_cmd   - X;
ERR_Y   = Y_cmd   - Y;
ERR_PHI = PHI_cmd - PHI;



% ===== X =====
X_cmd_dot = (X_cmd - X_cmd_pos)/dt ;
X_cmd_dotdot = (X_cmd_dot - X_cmd_dot_pos)/dt;

S_X = (ERR_X-ERR_X_pos)/dt+K*ERR_X;

if( abs(S_X)>=Slide_sat )
    Sat_X = sign(S_X);
else
    Sat_X =  S_X/Slide_sat;
end

X_all = X_cmd_dotdot + K*(ERR_X-ERR_X_pos)/dt - Sigma*Sat_X  + Y_dot*PHI_dot*(4*Iyw/(R^2)) ;

% ===== Y =====
Y_cmd_dot = (Y_cmd - Y_cmd_pos)*dt ;
Y_cmd_dotdot = (Y_cmd_dot - Y_cmd_dot_pos)*dt;

S_Y = (ERR_Y-ERR_Y_pos)/dt+K*ERR_Y;

if( abs(S_Y)>=Slide_sat )
    Sat_Y = sign(S_Y);
else
    Sat_Y =  S_Y/Slide_sat;
end

Y_all = Y_cmd_dotdot + K*(ERR_Y-ERR_Y_pos)/dt - Sigma*Sat_Y  - X_dot*PHI_dot*(4*Iyw/(R^2)) ;

% ===== PHI =====
PHI_cmd_dot = (PHI_cmd - PHI_cmd_pos)/dt ;
PHI_cmd_dotdot = (PHI_cmd_dot - PHI_cmd_dot_pos)/dt;

S_PHI = (ERR_PHI-ERR_PHI_pos)/dt + K*ERR_PHI;

if( abs(S_PHI)>=Slide_sat)
    Sat_PHI = sign(S_PHI);
else
    Sat_PHI =  S_PHI/Slide_sat;
end


PHI_all = PHI_cmd_dotdot + K*(ERR_PHI-ERR_PHI_pos)/dt -Sigma*Sat_PHI ;




% ===== TQC =====
a1 = mb + 4*mw  + 4*Iyw/(R^2);
a2 = Izb+ 4*Izw + 4*mw*(Lx^2+Ly^2) + 4*Iyw/(R^2)*((Lx+Ly)^2);

% === M1 ====
Buff_X   =  1/4*( cos(PHI)+sin(PHI) )*R*a1;
Buff_Y   = -1/4*( cos(PHI)-sin(PHI) )*R*a1;
Buff_PHI = -1/4/(Lx+Ly)*R*a2;

TQC1 = (Buff_X*X_all + Buff_Y*Y_all + Buff_PHI*PHI_all)/N;

% === M2 ====
Buff_X   =  1/4*( cos(PHI)-sin(PHI) )*R*a1;
Buff_Y   =  1/4*( cos(PHI)+sin(PHI) )*R*a1;
Buff_PHI =  1/4/(Lx+Ly)*R*a2;

TQC2 = (Buff_X*X_all + Buff_Y*Y_all + Buff_PHI*PHI_all)/N;

% === M3 ====
Buff_X   =  1/4*( cos(PHI)-sin(PHI) )*R*a1;
Buff_Y   =  1/4*( cos(PHI)+sin(PHI) )*R*a1;
Buff_PHI = -1/4/(Lx+Ly)*R*a2;

TQC3 = (Buff_X*X_all + Buff_Y*Y_all + Buff_PHI*PHI_all)/N;

% === M4 ====
Buff_X   =  1/4*( cos(PHI)+sin(PHI) )*R*a1;
Buff_Y   = -1/4*( cos(PHI)-sin(PHI) )*R*a1;
Buff_PHI =  1/4/(Lx+Ly)*R*a2;

TQC4 = (Buff_X*X_all + Buff_Y*Y_all + Buff_PHI*PHI_all)/N;





% TQC_to_Uc

U1 = TQC1/Kt;   %TQC1*Ra/Kt + w1*(Kb)^2;
U2 = TQC2/Kt;   %TQC2*Ra/Kt + w2*(Kb)^2;
U3 = TQC3/Kt;   %TQC3*Ra/Kt + w3*(Kb)^2;
U4 = TQC4/Kt;   %TQC4*Ra/Kt + w4*(Kb)^2;

if ( abs(U1)>MaxU )
    U1 = sign(U1)*MaxU;
end

if ( abs(U2)>MaxU )
    U2 = sign(U2)*MaxU;
end

if ( abs(U3)>MaxU )
    U3 = sign(U3)*MaxU;
end

if ( abs(U4)>MaxU )
    U4 = sign(U4)*MaxU;
end



%===== Recorder =====
X_cmd_pos = X_cmd;
Y_cmd_pos = Y_cmd;
PHI_cmd_pos = PHI_cmd;

X_cmd_dot_pos = X_cmd_dot;
Y_cmd_dot_pos = Y_cmd_dot;
PHI_cmd_dot_pos = PHI_cmd_dot;

ERR_X_pos   = ERR_X;
ERR_Y_pos   = ERR_Y;
ERR_PHI_pos = ERR_PHI;

== matlab function Mecanum_Mfunction_SM/Path_Planning/T_curve_phi/T_curve ==
  settings: updateMethod=DISCRETE  sampleTime=0.001
  data: A data_store_memory; Cmd_phi_output output; Vcmd_phi_output output; Final_phi input; TEST output; Final_phi_pos data_store_memory; Vcmd_phi data_store_memory; Accel_sign_phi data_store_memory; Need_Dis_phi data_store_memory; Need_Dis_phi_Buff data_store_memory; DeAccel_phi data_store_memory; Cmd_phi data_store_memory
function [Cmd_phi_output,Vcmd_phi_output,TEST]    = fcn(Final_phi)

%==== Ver 2 =====

global A;
global Final_phi_pos;
global Vcmd_phi;
global Accel_sign_phi;
global Need_Dis_phi;
global Need_Dis_phi_Buff;
global DeAccel_phi;
global Cmd_phi;

%===== Parameter=====
Max_Accel = pi/4;
Max_Velocity = pi/4;
Pos_Standard = 0.1;
dt = 0.001;

%=== CHECK Final Change? ===
if(Final_phi ~= Final_phi_pos)
    Need_Dis_phi = Final_phi - Cmd_phi;
    Need_Dis_phi_Buff =0;
    DeAccel_phi =0;
    
    %=== Direction Check ===
	if (Need_Dis_phi >0)
        Accel_sign_phi =  1;
	elseif (Need_Dis_phi <0)
		Accel_sign_phi = -1;
	else
		Accel_sign_phi =  0;
	end
end
    
Detime_phi = abs(Vcmd_phi/Max_Accel);

%===== DeAccel Cehck =====
     Buff = Need_Dis_phi_Buff + Vcmd_phi*Detime_phi + 1/2*(-1*Accel_sign_phi*Max_Accel)*Detime_phi*Detime_phi;
    
    if((Buff>Need_Dis_phi) && (Accel_sign_phi==1))
        DeAccel_phi = 1;
    elseif ((Buff<Need_Dis_phi) && (Accel_sign_phi==-1))
        DeAccel_phi = 1;
    else
        DeAccel_phi = 0;
    end
    
%===== Vel Cal =====
if(DeAccel_phi ==0)
    Vcmd_phi = Vcmd_phi + Accel_sign_phi * Max_Accel*dt;
elseif(DeAccel_phi ==1) 
    Vcmd_phi = Vcmd_phi - Accel_sign_phi * Max_Accel*dt;
    Buff = Vcmd_phi *Accel_sign_phi;
    if(Buff<0)
    Vcmd_phi = 0;
    end
end

%===== Max Vel Check =====

if(Vcmd_phi > Max_Velocity)
    Vcmd_phi = Max_Velocity;
elseif (Vcmd_phi < -Max_Velocity)
    Vcmd_phi = -Max_Velocity;
end


Cmd_phi = Cmd_phi + Vcmd_phi * dt;
Need_Dis_phi_Buff = Need_Dis_phi_Buff + Vcmd_phi*dt;
Final_phi_pos = Final_phi;

%===== Output =====
Cmd_phi_output  = Cmd_phi ;
Vcmd_phi_output = Vcmd_phi;

A = A+1;
TEST =A;

== matlab function Mecanum_Mfunction_SM/MATLAB Function ==
  data: X input; Delta_mu output; Y input; x_hole input; y_hole input
function Delta_mu = fcn(X, Y, x_hole, y_hole)

Dis = ((X - x_hole)^2 + (Y - y_hole)^2)^0.5;
if(Dis < 1)
    D = 1;
else
    D = 0;
end
Delta_mu = D;
